simulink model "quatConversion_th"  (R2018b)
settings: Solver=VariableStepAuto  StartTime=0.0  StopTime=0  RelTol=1e-3
values from neighbouring files (symbols this model uses):
  eulAng = 2*(rand(3,1)-0.5)*90    [quatConversion_ts.m]
libraries: eulAng2RotMat_ul x1, vectorNormalizer_ul x1, quat2EulerAng_ul x1, rotMat2Quat_ul x1
settings Model: Creator=mcobb  LastModifiedBy=mcobb

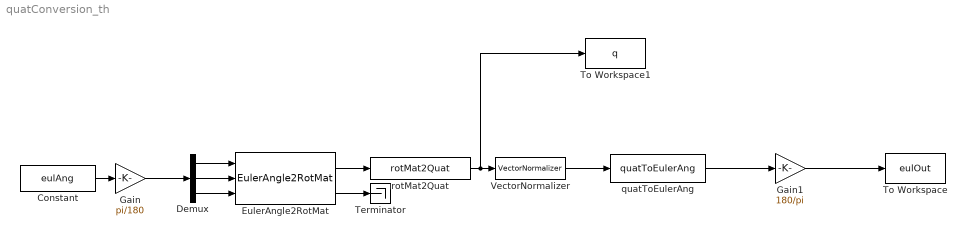
== system quatConversion_th ==
  Constant : Constant  Value=eulAng
  Demux : Demux  Outputs=3
  EulerAngle2RotMat : eulAng2RotMat_ul/EulerAngle2RotMat  SystemSampleTime=-1
  Gain : Gain  Gain=pi/180
  Gain1 : Gain  Gain=180/pi
  Terminator : Terminator
  To Workspace : ToWorkspace  VariableName=eulOut  SaveFormat=Timeseries  SampleTime=-1
  To Workspace1 : ToWorkspace  VariableName=q  SaveFormat=Timeseries  SampleTime=-1
  "VectorNormalizer " : vectorNormalizer_ul/VectorNormalizer   SystemSampleTime=-1
  quatToEulerAng : quat2EulerAng_ul/quatToEulerAng  SystemSampleTime=-1
  rotMat2Quat : rotMat2Quat_ul/rotMat2Quat  SystemSampleTime=-1
  wires:
  rotMat2Quat/1 -> To Workspace1/1, "VectorNormalizer "/1
  EulerAngle2RotMat/1 -> rotMat2Quat/1
  EulerAngle2RotMat/2 -> Terminator/1
  Demux/2 -> EulerAngle2RotMat/2
  Demux/1 -> EulerAngle2RotMat/1
  Demux/3 -> EulerAngle2RotMat/3
  Constant/1 -> Gain/1
  "VectorNormalizer "/1 -> quatToEulerAng/1
  Gain/1 -> Demux/1
  Gain1/1 -> To Workspace/1
  quatToEulerAng/1 -> Gain1/1
